simulink model "LUT_liver_pancreas_25"  (R2023b)
settings: Solver=FixedStepAuto  StartTime=0  StopTime=10.1  FixedStep=Timegap  RelTol=1e-3
model workspace (MAT data in the model file):
  T1_input = 1.34
(part 2 of 3)

== system LUT_liver_pancreas_25/If Action Subsystem6/If Action Subsystem1/If Action Subsystem6/If Action Subsystem3 ==
  In1 : Inport
  Action Port : ActionPort  ActionPortLabel=elseif( u1 >= 1.025)
  LUT 1.03RR : Lookup_n-D  NumberOfTableDimensions=1  BreakpointsForDimension1=[403.1578;512.2788;611.2464;710.3985;809.5013;908.5484;1007.552;1106.523;1205.471;1304.4;1403.315;1502.219;1601.114;1700.001;1798.878;1897.738;1996.552]  Table=[400;500;600;700;800;900;1000;1100;1200;1300;1400;1500;1600;1700;1800;1900;2000]  InternalRulePriority=Speed  RndMeth=Simplest
  Out1 : Outport
  wires:
  In1/1 -> LUT 1.03RR/1
  LUT 1.03RR/1 -> Out1/1

== system LUT_liver_pancreas_25/If Action Subsystem6/If Action Subsystem1/If Action Subsystem6/If Action Subsystem4 ==
  In1 : Inport
  Action Port : ActionPort  ActionPortLabel=elseif( u1 >= 1.035)
  LUT 1.04RR : Lookup_n-D  NumberOfTableDimensions=1  BreakpointsForDimension1=[403.058;512.1074;611.0037;710.0774;809.0975;908.0593;1006.976;1105.859;1204.716;1303.555;1402.38;1501.193;1599.996;1698.791;1797.577;1896.347;1995.079]  Table=[400;500;600;700;800;900;1000;1100;1200;1300;1400;1500;1600;1700;1800;1900;2000]  InternalRulePriority=Speed  RndMeth=Simplest
  Out1 : Outport
  wires:
  In1/1 -> LUT 1.04RR/1
  LUT 1.04RR/1 -> Out1/1

== system LUT_liver_pancreas_25/If Action Subsystem6/If Action Subsystem1/If Action Subsystem6/If Action Subsystem5 ==
  In1 : Inport
  Action Port : ActionPort  ActionPortLabel=elseif( u1 >= 1.055)
  LUT 1.06RR : Lookup_n-D  NumberOfTableDimensions=1  BreakpointsForDimension1=[402.866;511.7786;610.5383;709.461;808.3215;907.1183;1005.866;1104.578;1203.263;1301.927;1400.576;1499.212;1597.839;1696.456;1795.064;1893.659;1992.228]  Table=[400;500;600;700;800;900;1000;1100;1200;1300;1400;1500;1600;1700;1800;1900;2000]  InternalRulePriority=Speed  RndMeth=Simplest
  Out1 : Outport
  wires:
  In1/1 -> LUT 1.06RR/1
  LUT 1.06RR/1 -> Out1/1

== system LUT_liver_pancreas_25/If Action Subsystem6/If Action Subsystem1/If Action Subsystem6/If Action Subsystem6 ==
  In1 : Inport
  Action Port : ActionPort  ActionPortLabel=elseif( u1 >= 1.045)
  LUT 1.05RR : Lookup_n-D  NumberOfTableDimensions=1  BreakpointsForDimension1=[402.9608;511.9407;610.7678;709.765;808.7044;907.5827;1006.414;1105.21;1203.981;1302.731;1401.467;1500.191;1598.905;1697.61;1796.306;1894.988;1993.638]  Table=[400;500;600;700;800;900;1000;1100;1200;1300;1400;1500;1600;1700;1800;1900;2000]  InternalRulePriority=Speed  RndMeth=Simplest
  Out1 : Outport
  wires:
  In1/1 -> LUT 1.05RR/1
  LUT 1.05RR/1 -> Out1/1

== system LUT_liver_pancreas_25/If Action Subsystem6/If Action Subsystem1/If Action Subsystem6/If Action Subsystem7 ==
  In1 : Inport
  Action Port : ActionPort  ActionPortLabel=elseif( u1 >= 1.065)
  LUT 1.07RR : Lookup_n-D  NumberOfTableDimensions=1  BreakpointsForDimension1=[402.7736;511.6208;610.315;709.165;807.9485;906.6656;1005.332;1103.961;1202.562;1301.142;1399.706;1498.257;1596.797;1695.328;1793.85;1892.36;1990.847]  Table=[400;500;600;700;800;900;1000;1100;1200;1300;1400;1500;1600;1700;1800;1900;2000]  InternalRulePriority=Speed  RndMeth=Simplest
  Out1 : Outport
  wires:
  In1/1 -> LUT 1.07RR/1
  LUT 1.07RR/1 -> Out1/1

== system LUT_liver_pancreas_25/If Action Subsystem6/If Action Subsystem1/If Action Subsystem6/If Action Subsystem8 ==
  In1 : Inport
  Action Port : ActionPort  ActionPortLabel=elseif(u1 >= 1.075)
  LUT 1.08RR : Lookup_n-D  NumberOfTableDimensions=1  BreakpointsForDimension1=[402.6834;511.4673;610.0977;708.8767;807.585;906.2243;1004.811;1103.359;1201.878;1300.375;1398.855;1497.323;1595.779;1694.226;1792.664;1891.09;1989.496]  Table=[400;500;600;700;800;900;1000;1100;1200;1300;1400;1500;1600;1700;1800;1900;2000]  InternalRulePriority=Speed  RndMeth=Simplest
  Out1 : Outport
  wires:
  In1/1 -> LUT 1.08RR/1
  LUT 1.08RR/1 -> Out1/1

== system LUT_liver_pancreas_25/If Action Subsystem6/If Action Subsystem1/If Action Subsystem6/If Action Subsystem9 ==
  In1 : Inport
  Action Port : ActionPort  ActionPortLabel=if(u1 >= 1.085)
  LUT 1.09RR : Lookup_n-D  NumberOfTableDimensions=1  BreakpointsForDimension1=[402.5954;511.3177;609.886;708.5958;807.2308;905.7938;1004.302;1102.771;1201.21;1299.626;1398.025;1496.41;1594.784;1693.149;1791.504;1889.848;1988.174]  Table=[400;500;600;700;800;900;1000;1100;1200;1300;1400;1500;1600;1700;1800;1900;2000]  InternalRulePriority=Speed  RndMeth=Simplest
  Out1 : Outport
  wires:
  In1/1 -> LUT 1.09RR/1
  LUT 1.09RR/1 -> Out1/1

== system LUT_liver_pancreas_25/If Action Subsystem6/If Action Subsystem1/If Action Subsystem7/If Action Subsystem1 ==
  In1 : Inport
  Action Port : ActionPort  ActionPortLabel=elseif( u1 >= 1.215)
  LUT 1.22RR : Lookup_n-D  NumberOfTableDimensions=1  BreakpointsForDimension1=[401.6092;509.6767;607.5712;705.5178;803.3346;901.0436;998.6735;1096.246;1193.776;1291.274;1388.747;1486.201;1583.64;1681.066;1778.481;1875.887;1973.283]  Table=[400;500;600;700;800;900;1000;1100;1200;1300;1400;1500;1600;1700;1800;1900;2000]  InternalRulePriority=Speed  RndMeth=Simplest
  Out1 : Outport
  wires:
  In1/1 -> LUT 1.22RR/1
  LUT 1.22RR/1 -> Out1/1

== system LUT_liver_pancreas_25/If Action Subsystem6/If Action Subsystem1/If Action Subsystem7/If Action Subsystem10 ==
  In1 : Inport
  Action Port : ActionPort  ActionPortLabel=elseif( u1 >= 1.205)
  LUT 1.21RR : Lookup_n-D  NumberOfTableDimensions=1  BreakpointsForDimension1=[401.6763;509.7858;607.7244;705.7218;803.5935;901.3603;999.0498;1096.683;1194.275;1291.836;1389.373;1486.891;1584.394;1681.884;1779.364;1876.834;1974.294]  Table=[400;500;600;700;800;900;1000;1100;1200;1300;1400;1500;1600;1700;1800;1900;2000]  InternalRulePriority=Speed  RndMeth=Simplest
  Out1 : Outport
  wires:
  In1/1 -> LUT 1.21RR/1
  LUT 1.21RR/1 -> Out1/1

== system LUT_liver_pancreas_25/If Action Subsystem6/If Action Subsystem1/If Action Subsystem7/If Action Subsystem2 ==
  In1 : Inport
  Action Port : ActionPort  ActionPortLabel=else
  LUT 1.20RR : Lookup_n-D  NumberOfTableDimensions=1  BreakpointsForDimension1=[401.7447;509.8975;607.8813;705.9306;803.8585;901.6842;999.4346;1097.13;1194.785;1292.41;1390.012;1487.594;1585.163;1682.719;1780.264;1877.8;1975.326]  Table=[400;500;600;700;800;900;1000;1100;1200;1300;1400;1500;1600;1700;1800;1900;2000]  InternalRulePriority=Speed  RndMeth=Simplest
  Out1 : Outport
  wires:
  In1/1 -> LUT 1.20RR/1
  LUT 1.20RR/1 -> Out1/1

== system LUT_liver_pancreas_25/If Action Subsystem6/If Action Subsystem1/If Action Subsystem7/If Action Subsystem3 ==
  In1 : Inport
  Action Port : ActionPort  ActionPortLabel=elseif( u1 >= 1.225)
  LUT 1.23RR : Lookup_n-D  NumberOfTableDimensions=1  BreakpointsForDimension1=[401.5433;509.5699;607.4215;705.3185;803.0815;900.7339;998.3054;1095.818;1193.287;1290.723;1388.135;1485.526;1582.902;1680.265;1777.616;1874.958;1972.291]  Table=[400;500;600;700;800;900;1000;1100;1200;1300;1400;1500;1600;1700;1800;1900;2000]  InternalRulePriority=Speed  RndMeth=Simplest
  Out1 : Outport
  wires:
  In1/1 -> LUT 1.23RR/1
  LUT 1.23RR/1 -> Out1/1

== system LUT_liver_pancreas_25/If Action Subsystem6/If Action Subsystem1/If Action Subsystem7/If Action Subsystem4 ==
  In1 : Inport
  Action Port : ActionPort  ActionPortLabel=elseif( u1 >= 1.235)
  LUT 1.24RR : Lookup_n-D  NumberOfTableDimensions=1  BreakpointsForDimension1=[401.4785;509.4655;607.2752;705.1238;802.8342;900.4312;997.9452;1095.399;1192.808;1290.184;1387.534;1484.864;1582.178;1679.479;1776.768;1874.048;1971.318]  Table=[400;500;600;700;800;900;1000;1100;1200;1300;1400;1500;1600;1700;1800;1900;2000]  InternalRulePriority=Speed  RndMeth=Simplest
  Out1 : Outport
  wires:
  In1/1 -> LUT 1.24RR/1
  LUT 1.24RR/1 -> Out1/1

== system LUT_liver_pancreas_25/If Action Subsystem6/If Action Subsystem1/If Action Subsystem7/If Action Subsystem5 ==
  In1 : Inport
  Action Port : ActionPort  ActionPortLabel=elseif( u1 >= 1.255)
  LUT 1.26RR : Lookup_n-D  NumberOfTableDimensions=1  BreakpointsForDimension1=[401.3524;509.2634;606.9926;704.7476;802.3561;899.8455;997.2481;1094.588;1191.881;1289.139;1386.37;1483.58;1580.774;1677.953;1775.121;1872.279;1969.428]  Table=[400;500;600;700;800;900;1000;1100;1200;1300;1400;1500;1600;1700;1800;1900;2000]  InternalRulePriority=Speed  RndMeth=Simplest
  Out1 : Outport
  wires:
  In1/1 -> LUT 1.26RR/1
  LUT 1.26RR/1 -> Out1/1

== system LUT_liver_pancreas_25/If Action Subsystem6/If Action Subsystem1/If Action Subsystem7/If Action Subsystem6 ==
  In1 : Inport
  Action Port : ActionPort  ActionPortLabel=elseif( u1 >= 1.245)
  LUT 1.25RR : Lookup_n-D  NumberOfTableDimensions=1  BreakpointsForDimension1=[401.4149;509.3633;607.1323;704.9335;802.5924;900.1351;997.5929;1094.989;1192.34;1289.656;1386.946;1484.216;1581.469;1678.709;1775.937;1873.155;1970.364]  Table=[400;500;600;700;800;900;1000;1100;1200;1300;1400;1500;1600;1700;1800;1900;2000]  InternalRulePriority=Speed  RndMeth=Simplest
  Out1 : Outport
  wires:
  In1/1 -> LUT 1.25RR/1
  LUT 1.25RR/1 -> Out1/1

== system LUT_liver_pancreas_25/If Action Subsystem6/If Action Subsystem1/If Action Subsystem7/If Action Subsystem7 ==
  In1 : Inport
  Action Port : ActionPort  ActionPortLabel=elseif( u1 >= 1.265)
  LUT 1.27RR : Lookup_n-D  NumberOfTableDimensions=1  BreakpointsForDimension1=[401.291;509.1656;606.856;704.5658;802.125;899.5622;996.9107;1094.195;1191.431;1288.632;1385.806;1482.957;1580.092;1677.213;1774.322;1871.42;1968.51]  Table=[400;500;600;700;800;900;1000;1100;1200;1300;1400;1500;1600;1700;1800;1900;2000]  InternalRulePriority=Speed  RndMeth=Simplest
  Out1 : Outport
  wires:
  In1/1 -> LUT 1.27RR/1
  LUT 1.27RR/1 -> Out1/1

== system LUT_liver_pancreas_25/If Action Subsystem6/If Action Subsystem1/If Action Subsystem7/If Action Subsystem8 ==
  In1 : Inport
  Action Port : ActionPort  ActionPortLabel=elseif(u1 >= 1.275)
  LUT 1.28RR : Lookup_n-D  NumberOfTableDimensions=1  BreakpointsForDimension1=[401.2306;509.0698;606.7226;704.3882;801.899;899.2851;996.5805;1093.81;1190.991;1288.136;1385.252;1482.347;1579.424;1676.486;1773.537;1870.577;1967.608]  Table=[400;500;600;700;800;900;1000;1100;1200;1300;1400;1500;1600;1700;1800;1900;2000]  InternalRulePriority=Speed  RndMeth=Simplest
  Out1 : Outport
  wires:
  In1/1 -> LUT 1.28RR/1
  LUT 1.28RR/1 -> Out1/1

== system LUT_liver_pancreas_25/If Action Subsystem6/If Action Subsystem1/If Action Subsystem7/If Action Subsystem9 ==
  In1 : Inport
  Action Port : ActionPort  ActionPortLabel=if(u1 >= 1.285)
  LUT 1.29RR : Lookup_n-D  NumberOfTableDimensions=1  BreakpointsForDimension1=[401.1711;508.9761;606.5921;704.2145;801.678;899.014;996.2573;1093.433;1190.56;1287.649;1384.71;1481.748;1578.768;1675.774;1772.767;1869.751;1966.724]  Table=[400;500;600;700;800;900;1000;1100;1200;1300;1400;1500;1600;1700;1800;1900;2000]  InternalRulePriority=Speed  RndMeth=Simplest
  Out1 : Outport
  wires:
  In1/1 -> LUT 1.29RR/1
  LUT 1.29RR/1 -> Out1/1

== system LUT_liver_pancreas_25/If Action Subsystem6/If Action Subsystem1/If Action Subsystem8/If Action Subsystem1 ==
  In1 : Inport
  Action Port : ActionPort  ActionPortLabel=elseif( u1 >= 1.315)
  LUT 1.32RR : Lookup_n-D  NumberOfTableDimensions=1  BreakpointsForDimension1=[400.9985;508.7063;606.2176;703.7164;801.0438;898.2352;995.328;1092.349;1189.318;1286.247;1383.146;1480.021;1576.876;1673.717;1770.544;1867.361;1964.168]  Table=[400;500;600;700;800;900;1000;1100;1200;1300;1400;1500;1600;1700;1800;1900;2000]  InternalRulePriority=Speed  RndMeth=Simplest
  Out1 : Outport
  wires:
  In1/1 -> LUT 1.32RR/1
  LUT 1.32RR/1 -> Out1/1

== system LUT_liver_pancreas_25/If Action Subsystem6/If Action Subsystem1/If Action Subsystem8/If Action Subsystem10 ==
  In1 : Inport
  Action Port : ActionPort  ActionPortLabel=elseif( u1 >= 1.305)
  LUT 1.31RR : Lookup_n-D  NumberOfTableDimensions=1  BreakpointsForDimension1=[401.0551;508.7943;606.3397;703.8787;801.2505;898.4892;995.6313;1092.703;1189.724;1286.705;1383.657;1480.585;1577.495;1674.389;1771.272;1868.143;1965.004]  Table=[400;500;600;700;800;900;1000;1100;1200;1300;1400;1500;1600;1700;1800;1900;2000]  InternalRulePriority=Speed  RndMeth=Simplest
  Out1 : Outport
  wires:
  In1/1 -> LUT 1.31RR/1
  LUT 1.31RR/1 -> Out1/1

== system LUT_liver_pancreas_25/If Action Subsystem6/If Action Subsystem1/If Action Subsystem8/If Action Subsystem2 ==
  In1 : Inport
  Action Port : ActionPort  ActionPortLabel=else
  LUT 1.30RR : Lookup_n-D  NumberOfTableDimensions=1  BreakpointsForDimension1=[401.1126;508.8843;606.4645;704.0447;801.4619;898.7488;995.941;1093.065;1190.137;1287.172;1384.178;1481.161;1578.125;1675.075;1772.012;1868.939;1965.856]  Table=[400;500;600;700;800;900;1000;1100;1200;1300;1400;1500;1600;1700;1800;1900;2000]  InternalRulePriority=Speed  RndMeth=Simplest
  Out1 : Outport
  wires:
  In1/1 -> LUT 1.30RR/1
  LUT 1.30RR/1 -> Out1/1

== system LUT_liver_pancreas_25/If Action Subsystem6/If Action Subsystem1/If Action Subsystem8/If Action Subsystem3 ==
  In1 : Inport
  Action Port : ActionPort  ActionPortLabel=elseif( u1 >= 1.325)
  LUT 1.33RR : Lookup_n-D  NumberOfTableDimensions=1  BreakpointsForDimension1=[400.9427;508.62;606.0983;703.5577;800.8415;897.9866;995.0311;1092.003;1188.921;1285.798;1382.645;1479.467;1576.27;1673.057;1769.831;1866.594;1963.347]  Table=[400;500;600;700;800;900;1000;1100;1200;1300;1400;1500;1600;1700;1800;1900;2000]  InternalRulePriority=Speed  RndMeth=Simplest
  Out1 : Outport
  wires:
  In1/1 -> LUT 1.33RR/1
  LUT 1.33RR/1 -> Out1/1

== system LUT_liver_pancreas_25/If Action Subsystem6/If Action Subsystem1/If Action Subsystem8/If Action Subsystem4 ==
  In1 : Inport
  Action Port : ActionPort  ActionPortLabel=elseif( u1 >= 1.335)
  LUT 1.34RR : Lookup_n-D  NumberOfTableDimensions=1  BreakpointsForDimension1=[400.8878;508.5354;605.9815;703.4024;800.6436;897.7433;994.7404;1091.663;1188.531;1285.358;1382.153;1478.924;1575.674;1672.409;1769.131;1865.841;1962.541]  Table=[400;500;600;700;800;900;1000;1100;1200;1300;1400;1500;1600;1700;1800;1900;2000]  InternalRulePriority=Speed  RndMeth=Simplest
  Out1 : Outport
  wires:
  In1/1 -> LUT 1.34RR/1
  LUT 1.34RR/1 -> Out1/1

== system LUT_liver_pancreas_25/If Action Subsystem6/If Action Subsystem1/If Action Subsystem8/If Action Subsystem5 ==
  In1 : Inport
  Action Port : ActionPort  ActionPortLabel=elseif( u1 >= 1.355)
  LUT 1.36RR : Lookup_n-D  NumberOfTableDimensions=1  BreakpointsForDimension1=[400.7805;508.3714;605.7554;703.102;800.2606;897.272;994.1769;1091.005;1187.775;1284.503;1381.198;1477.868;1574.517;1671.149;1767.768;1864.375;1960.972]  Table=[400;500;600;700;800;900;1000;1100;1200;1300;1400;1500;1600;1700;1800;1900;2000]  InternalRulePriority=Speed  RndMeth=Simplest
  Out1 : Outport
  wires:
  In1/1 -> LUT 1.36RR/1
  LUT 1.36RR/1 -> Out1/1

== system LUT_liver_pancreas_25/If Action Subsystem6/If Action Subsystem1/If Action Subsystem8/If Action Subsystem6 ==
  In1 : Inport
  Action Port : ActionPort  ActionPortLabel=elseif( u1 >= 1.345)
  LUT 1.35RR : Lookup_n-D  NumberOfTableDimensions=1  BreakpointsForDimension1=[400.8337;508.4526;605.8672;703.2505;800.4501;897.5052;994.4557;1091.331;1188.15;1284.926;1381.671;1478.391;1575.09;1671.773;1768.443;1865.101;1961.75]  Table=[400;500;600;700;800;900;1000;1100;1200;1300;1400;1500;1600;1700;1800;1900;2000]  InternalRulePriority=Speed  RndMeth=Simplest
  Out1 : Outport
  wires:
  In1/1 -> LUT 1.35RR/1
  LUT 1.35RR/1 -> Out1/1

== system LUT_liver_pancreas_25/If Action Subsystem6/If Action Subsystem1/If Action Subsystem8/If Action Subsystem7 ==
  In1 : Inport
  Action Port : ActionPort  ActionPortLabel=elseif( u1 >= 1.365)
  LUT 1.37RR : Lookup_n-D  NumberOfTableDimensions=1  BreakpointsForDimension1=[400.728;508.2918;605.646;702.9566;800.0753;897.0438;993.9039;1090.685;1187.409;1284.088;1380.735;1477.355;1573.954;1670.537;1767.105;1863.662;1960.209]  Table=[400;500;600;700;800;900;1000;1100;1200;1300;1400;1500;1600;1700;1800;1900;2000]  InternalRulePriority=Speed  RndMeth=Simplest
  Out1 : Outport
  wires:
  In1/1 -> LUT 1.37RR/1
  LUT 1.37RR/1 -> Out1/1

== system LUT_liver_pancreas_25/If Action Subsystem6/If Action Subsystem1/If Action Subsystem8/If Action Subsystem8 ==
  In1 : Inport
  Action Port : ActionPort  ActionPortLabel=elseif(u1 >= 1.375)
  LUT 1.38RR : Lookup_n-D  NumberOfTableDimensions=1  BreakpointsForDimension1=[400.6763;508.2137;605.539;702.8145;799.8939;896.8204;993.6364;1090.372;1187.049;1283.682;1380.28;1476.852;1573.402;1669.936;1766.455;1862.962;1959.459]  Table=[400;500;600;700;800;900;1000;1100;1200;1300;1400;1500;1600;1700;1800;1900;2000]  InternalRulePriority=Speed  RndMeth=Simplest
  Out1 : Outport
  wires:
  In1/1 -> LUT 1.38RR/1
  LUT 1.38RR/1 -> Out1/1

== system LUT_liver_pancreas_25/If Action Subsystem6/If Action Subsystem1/If Action Subsystem8/If Action Subsystem9 ==
  In1 : Inport
  Action Port : ActionPort  ActionPortLabel=if(u1 >= 1.385)
  LUT 1.39RR : Lookup_n-D  NumberOfTableDimensions=1  BreakpointsForDimension1=[400.6253;508.1372;605.4342;702.6754;799.7164;896.6017;993.3744;1090.066;1186.697;1283.283;1379.834;1476.358;1572.86;1669.345;1765.816;1862.275;1958.723]  Table=[400;500;600;700;800;900;1000;1100;1200;1300;1400;1500;1600;1700;1800;1900;2000]  InternalRulePriority=Speed  RndMeth=Simplest
  Out1 : Outport
  wires:
  In1/1 -> LUT 1.39RR/1
  LUT 1.39RR/1 -> Out1/1

== system LUT_liver_pancreas_25/If Action Subsystem6/If Action Subsystem1/If Action Subsystem9/If Action Subsystem1 ==
  In1 : Inport
  Action Port : ActionPort  ActionPortLabel=elseif( u1 >= 1.415)
  LUT 1.42RR : Lookup_n-D  NumberOfTableDimensions=1  BreakpointsForDimension1=[400.4767;507.9164;605.133;702.2758;799.2063;895.9725;992.6201;1089.182;1185.68;1282.131;1378.545;1474.931;1571.293;1667.638;1763.967;1860.284;1956.59]  Table=[400;500;600;700;800;900;1000;1100;1200;1300;1400;1500;1600;1700;1800;1900;2000]  InternalRulePriority=Speed  RndMeth=Simplest
  Out1 : Outport
  wires:
  In1/1 -> LUT 1.42RR/1
  LUT 1.42RR/1 -> Out1/1

== system LUT_liver_pancreas_25/If Action Subsystem6/If Action Subsystem1/If Action Subsystem9/If Action Subsystem10 ==
  In1 : Inport
  Action Port : ActionPort  ActionPortLabel=elseif( u1 >= 1.405)
  LUT 1.41RR : Lookup_n-D  NumberOfTableDimensions=1  BreakpointsForDimension1=[400.5255;507.9886;605.2312;702.4061;799.3727;896.1778;992.8664;1089.471;1186.012;1282.507;1378.966;1475.397;1571.806;1668.197;1764.572;1860.936;1957.288]  Table=[400;500;600;700;800;900;1000;1100;1200;1300;1400;1500;1600;1700;1800;1900;2000]  InternalRulePriority=Speed  RndMeth=Simplest
  Out1 : Outport
  wires:
  In1/1 -> LUT 1.41RR/1
  LUT 1.41RR/1 -> Out1/1

== system LUT_liver_pancreas_25/If Action Subsystem6/If Action Subsystem1/If Action Subsystem9/If Action Subsystem2 ==
  In1 : Inport
  Action Port : ActionPort  ActionPortLabel=else
  LUT 1.40RR : Lookup_n-D  NumberOfTableDimensions=1  BreakpointsForDimension1=[400.5751;508.0622;605.3316;702.5393;799.5427;896.3875;993.1178;1089.765;1186.351;1282.891;1379.396;1475.873;1572.328;1668.766;1765.189;1861.599;1957.999]  Table=[400;500;600;700;800;900;1000;1100;1200;1300;1400;1500;1600;1700;1800;1900;2000]  InternalRulePriority=Speed  RndMeth=Simplest
  Out1 : Outport
  wires:
  In1/1 -> LUT 1.40RR/1
  LUT 1.40RR/1 -> Out1/1

== system LUT_liver_pancreas_25/If Action Subsystem6/If Action Subsystem1/If Action Subsystem9/If Action Subsystem3 ==
  In1 : Inport
  Action Port : ActionPort  ActionPortLabel=elseif( u1 >= 1.425)
  LUT 1.43RR : Lookup_n-D  NumberOfTableDimensions=1  BreakpointsForDimension1=[400.4285;507.8455;605.0367;702.1483;799.0434;895.7714;992.3788;1088.899;1185.354;1281.762;1378.131;1474.472;1570.79;1667.089;1763.373;1859.643;1955.903]  Table=[400;500;600;700;800;900;1000;1100;1200;1300;1400;1500;1600;1700;1800;1900;2000]  InternalRulePriority=Speed  RndMeth=Simplest
  Out1 : Outport
  wires:
  In1/1 -> LUT 1.43RR/1
  LUT 1.43RR/1 -> Out1/1

== system LUT_liver_pancreas_25/If Action Subsystem6/If Action Subsystem1/If Action Subsystem9/If Action Subsystem4 ==
  In1 : Inport
  Action Port : ActionPort  ActionPortLabel=elseif( u1 >= 1.435)
  LUT 1.44RR : Lookup_n-D  NumberOfTableDimensions=1  BreakpointsForDimension1=[400.381;507.776;604.9425;702.0235;798.884;895.5745;992.1424;1088.621;1185.035;1281.399;1377.726;1474.022;1570.296;1666.55;1762.789;1859.014;1955.229]  Table=[400;500;600;700;800;900;1000;1100;1200;1300;1400;1500;1600;1700;1800;1900;2000]  InternalRulePriority=Speed  RndMeth=Simplest
  Out1 : Outport
  wires:
  In1/1 -> LUT 1.44RR/1
  LUT 1.44RR/1 -> Out1/1

== system LUT_liver_pancreas_25/If Action Subsystem6/If Action Subsystem1/If Action Subsystem9/If Action Subsystem5 ==
  In1 : Inport
  Action Port : ActionPort  ActionPortLabel=elseif( u1 >= 1.455)
  LUT 1.46RR : Lookup_n-D  NumberOfTableDimensions=1  BreakpointsForDimension1=[400.2879;507.6409;604.76;701.7818;798.5751;895.1928;991.6838;1088.083;1184.414;1280.695;1376.936;1473.147;1569.333;1665.5;1761.651;1857.788;1953.914]  Table=[400;500;600;700;800;900;1000;1100;1200;1300;1400;1500;1600;1700;1800;1900;2000]  InternalRulePriority=Speed  RndMeth=Simplest
  Out1 : Outport
  wires:
  In1/1 -> LUT 1.46RR/1
  LUT 1.46RR/1 -> Out1/1

== system LUT_liver_pancreas_25/If Action Subsystem6/If Action Subsystem1/If Action Subsystem9/If Action Subsystem6 ==
  In1 : Inport
  Action Port : ActionPort  ActionPortLabel=elseif( u1 >= 1.445)
  LUT 1.45RR : Lookup_n-D  NumberOfTableDimensions=1  BreakpointsForDimension1=[400.3341;507.7078;604.8503;701.9014;798.7279;895.3816;991.9107;1088.35;1184.722;1281.044;1377.327;1473.581;1569.81;1666.02;1762.215;1858.396;1954.566]  Table=[400;500;600;700;800;900;1000;1100;1200;1300;1400;1500;1600;1700;1800;1900;2000]  InternalRulePriority=Speed  RndMeth=Simplest
  Out1 : Outport
  wires:
  In1/1 -> LUT 1.45RR/1
  LUT 1.45RR/1 -> Out1/1

== system LUT_liver_pancreas_25/If Action Subsystem6/If Action Subsystem1/If Action Subsystem9/If Action Subsystem7 ==
  In1 : Inport
  Action Port : ActionPort  ActionPortLabel=elseif( u1 >= 1.465)
  LUT 1.47RR : Lookup_n-D  NumberOfTableDimensions=1  BreakpointsForDimension1=[400.2422;507.5752;604.6715;701.6648;798.4255;895.0078;991.4613;1087.822;1184.113;1280.353;1376.552;1472.721;1568.865;1664.989;1761.097;1857.191;1953.274]  Table=[400;500;600;700;800;900;1000;1100;1200;1300;1400;1500;1600;1700;1800;1900;2000]  InternalRulePriority=Speed  RndMeth=Simplest
  Out1 : Outport
  wires:
  In1/1 -> LUT 1.47RR/1
  LUT 1.47RR/1 -> Out1/1

== system LUT_liver_pancreas_25/If Action Subsystem6/If Action Subsystem1/If Action Subsystem9/If Action Subsystem8 ==
  In1 : Inport
  Action Port : ActionPort  ActionPortLabel=elseif(u1 >= 1.475)
  LUT 1.48RR : Lookup_n-D  NumberOfTableDimensions=1  BreakpointsForDimension1=[400.1972;507.5108;604.5849;701.5503;798.2791;894.8266;991.2434;1087.565;1183.817;1280.017;1376.176;1472.303;1568.405;1664.487;1760.553;1856.604;1952.644]  Table=[400;500;600;700;800;900;1000;1100;1200;1300;1400;1500;1600;1700;1800;1900;2000]  InternalRulePriority=Speed  RndMeth=Simplest
  Out1 : Outport
  wires:
  In1/1 -> LUT 1.48RR/1
  LUT 1.48RR/1 -> Out1/1

== system LUT_liver_pancreas_25/If Action Subsystem6/If Action Subsystem1/If Action Subsystem9/If Action Subsystem9 ==
  In1 : Inport
  Action Port : ActionPort  ActionPortLabel=if(u1 >= 1.485)
  LUT 1.49RR : Lookup_n-D  NumberOfTableDimensions=1  BreakpointsForDimension1=[400.1527;507.4475;604.5;701.4382;798.1357;894.6491;991.0298;1087.314;1183.527;1279.687;1375.806;1471.893;1567.954;1663.994;1760.018;1856.028;1952.025]  Table=[400;500;600;700;800;900;1000;1100;1200;1300;1400;1500;1600;1700;1800;1900;2000]  InternalRulePriority=Speed  RndMeth=Simplest
  Out1 : Outport
  wires:
  In1/1 -> LUT 1.49RR/1
  LUT 1.49RR/1 -> Out1/1

== system LUT_liver_pancreas_25/If Action Subsystem6/If Action Subsystem2/If Action Subsystem5/If Action Subsystem1 ==
  In1 : Inport
  Action Port : ActionPort  ActionPortLabel=elseif( u1 >= 1.615)
  LUT 1.62RR : Lookup_n-D  NumberOfTableDimensions=1  BreakpointsForDimension1=[399.6228;506.7204;603.542;700.1784;796.523;892.6467;988.6108;1084.459;1180.221;1275.919;1371.567;1467.176;1562.753;1658.306;1753.839;1849.355;1944.857]  Table=[400;500;600;700;800;900;1000;1100;1200;1300;1400;1500;1600;1700;1800;1900;2000]  InternalRulePriority=Speed  RndMeth=Simplest
  Out1 : Outport
  wires:
  In1/1 -> LUT 1.62RR/1
  LUT 1.62RR/1 -> Out1/1

== system LUT_liver_pancreas_25/If Action Subsystem6/If Action Subsystem2/If Action Subsystem5/If Action Subsystem10 ==
  In1 : Inport
  Action Port : ActionPort  ActionPortLabel=elseif( u1>= 1.605)
  LUT 1.61RR : Lookup_n-D  NumberOfTableDimensions=1  BreakpointsForDimension1=[399.6606;506.7706;603.607;700.2634;796.632;892.7824;988.7753;1084.654;1180.448;1276.178;1371.858;1467.501;1563.113;1658.7;1754.268;1849.818;1945.355]  Table=[400;500;600;700;800;900;1000;1100;1200;1300;1400;1500;1600;1700;1800;1900;2000]  InternalRulePriority=Speed  RndMeth=Simplest
  Out1 : Outport
  wires:
  In1/1 -> LUT 1.61RR/1
  LUT 1.61RR/1 -> Out1/1

== system LUT_liver_pancreas_25/If Action Subsystem6/If Action Subsystem2/If Action Subsystem5/If Action Subsystem2 ==
  In1 : Inport
  Action Port : ActionPort  ActionPortLabel=else
  LUT 1.60RR : Lookup_n-D  NumberOfTableDimensions=1  BreakpointsForDimension1=[399.699;506.8217;603.6734;700.3504;796.7433;892.9209;988.9432;1084.853;1180.678;1276.441;1372.156;1467.832;1563.479;1659.101;1754.703;1850.289;1945.862]  Table=[400;500;600;700;800;900;1000;1100;1200;1300;1400;1500;1600;1700;1800;1900;2000]  InternalRulePriority=Speed  RndMeth=Simplest
  Out1 : Outport
  wires:
  In1/1 -> LUT 1.60RR/1
  LUT 1.60RR/1 -> Out1/1

== system LUT_liver_pancreas_25/If Action Subsystem6/If Action Subsystem2/If Action Subsystem5/If Action Subsystem3 ==
  In1 : Inport
  Action Port : ActionPort  ActionPortLabel=elseif( u1 >= 1.625)
  LUT 1.63RR : Lookup_n-D  NumberOfTableDimensions=1  BreakpointsForDimension1=[399.5853;506.671;603.4782;700.095;796.4163;892.5137;988.4495;1084.268;1179.999;1275.665;1371.28;1466.856;1562.4;1657.919;1753.418;1848.899;1944.366]  Table=[400;500;600;700;800;900;1000;1100;1200;1300;1400;1500;1600;1700;1800;1900;2000]  InternalRulePriority=Speed  RndMeth=Simplest
  Out1 : Outport
  wires:
  In1/1 -> LUT 1.63RR/1
  LUT 1.63RR/1 -> Out1/1

== system LUT_liver_pancreas_25/If Action Subsystem6/If Action Subsystem2/If Action Subsystem5/If Action Subsystem4 ==
  In1 : Inport
  Action Port : ActionPort  ActionPortLabel=elseif( u1 >= 1.635)
  LUT 1.64RR : Lookup_n-D  NumberOfTableDimensions=1  BreakpointsForDimension1=[399.5483;506.6225;603.4157;700.0135;796.3117;892.3834;988.2914;1084.08;1179.781;1275.415;1370.998;1466.542;1562.053;1657.538;1753.003;1848.451;1943.883]  Table=[400;500;600;700;800;900;1000;1100;1200;1300;1400;1500;1600;1700;1800;1900;2000]  InternalRulePriority=Speed  RndMeth=Simplest
  Out1 : Outport
  wires:
  In1/1 -> LUT 1.64RR/1
  LUT 1.64RR/1 -> Out1/1

== system LUT_liver_pancreas_25/If Action Subsystem6/If Action Subsystem2/If Action Subsystem5/If Action Subsystem5 ==
  In1 : Inport
  Action Port : ActionPort  ActionPortLabel=elseif( u1 >= 1.655)
  LUT 1.66RR : Lookup_n-D  NumberOfTableDimensions=1  BreakpointsForDimension1=[399.4756;506.5279;603.2945;699.8554;796.1092;892.1308;987.9845;1083.716;1179.357;1274.93;1370.45;1465.929;1561.376;1656.796;1752.195;1847.575;1942.941]  Table=[400;500;600;700;800;900;1000;1100;1200;1300;1400;1500;1600;1700;1800;1900;2000]  InternalRulePriority=Speed  RndMeth=Simplest
  Out1 : Outport
  wires:
  In1/1 -> LUT 1.66RR/1
  LUT 1.66RR/1 -> Out1/1

== system LUT_liver_pancreas_25/If Action Subsystem6/If Action Subsystem2/If Action Subsystem5/If Action Subsystem6 ==
  In1 : Inport
  Action Port : ActionPort  ActionPortLabel=elseif( u1 >= 1.645)
  LUT 1.65RR : Lookup_n-D  NumberOfTableDimensions=1  BreakpointsForDimension1=[399.5117;506.5748;603.3545;699.9336;796.2094;892.2558;988.1364;1083.896;1179.567;1275.17;1370.722;1466.233;1561.711;1657.164;1752.596;1848.009;1943.409]  Table=[400;500;600;700;800;900;1000;1100;1200;1300;1400;1500;1600;1700;1800;1900;2000]  InternalRulePriority=Speed  RndMeth=Simplest
  Out1 : Outport
  wires:
  In1/1 -> LUT 1.65RR/1
  LUT 1.65RR/1 -> Out1/1

== system LUT_liver_pancreas_25/If Action Subsystem6/If Action Subsystem2/If Action Subsystem5/If Action Subsystem7 ==
  In1 : Inport
  Action Port : ActionPort  ActionPortLabel=elseif( u1 >= 1.665)
  LUT 1.67RR : Lookup_n-D  NumberOfTableDimensions=1  BreakpointsForDimension1=[399.4398;506.4817;603.2356;699.7788;796.0111;892.0083;987.8356;1083.539;1179.151;1274.694;1370.183;1465.631;1561.046;1656.434;1751.8;1847.148;1942.482]  Table=[400;500;600;700;800;900;1000;1100;1200;1300;1400;1500;1600;1700;1800;1900;2000]  InternalRulePriority=Speed  RndMeth=Simplest
  Out1 : Outport
  wires:
  In1/1 -> LUT 1.67RR/1
  LUT 1.67RR/1 -> Out1/1

== system LUT_liver_pancreas_25/If Action Subsystem6/If Action Subsystem2/If Action Subsystem5/If Action Subsystem8 ==
  In1 : Inport
  Action Port : ActionPort  ActionPortLabel=elseif(u1 >= 1.675)
  LUT 1.68RR : Lookup_n-D  NumberOfTableDimensions=1  BreakpointsForDimension1=[399.4045;506.4364;603.1779;699.7038;795.915;891.8883;987.6896;1083.366;1178.949;1274.462;1369.921;1465.338;1560.722;1656.078;1751.412;1846.728;1942.029]  Table=[400;500;600;700;800;900;1000;1100;1200;1300;1400;1500;1600;1700;1800;1900;2000]  InternalRulePriority=Speed  RndMeth=Simplest
  Out1 : Outport
  wires:
  In1/1 -> LUT 1.68RR/1
  LUT 1.68RR/1 -> Out1/1

== system LUT_liver_pancreas_25/If Action Subsystem6/If Action Subsystem2/If Action Subsystem5/If Action Subsystem9 ==
  In1 : Inport
  Action Port : ActionPort  ActionPortLabel=if(u1 >= 1.685)
  LUT 1.69RR : Lookup_n-D  NumberOfTableDimensions=1  BreakpointsForDimension1=[399.3695;506.3918;603.1214;699.6304;795.8209;891.7708;987.5466;1083.196;1178.75;1274.234;1369.664;1465.05;1560.403;1655.728;1751.031;1846.315;1941.584]  Table=[400;500;600;700;800;900;1000;1100;1200;1300;1400;1500;1600;1700;1800;1900;2000]  InternalRulePriority=Speed  RndMeth=Simplest
  Out1 : Outport
  wires:
  In1/1 -> LUT 1.69RR/1
  LUT 1.69RR/1 -> Out1/1

== system LUT_liver_pancreas_25/If Action Subsystem6/If Action Subsystem2/If Action Subsystem6/If Action Subsystem1 ==
  In1 : Inport
  Action Port : ActionPort  ActionPortLabel=elseif( u1 >= 1.515)
  LUT 1.52RR : Lookup_n-D  NumberOfTableDimensions=1  BreakpointsForDimension1=[400.0228;507.2644;604.2558;701.1159;797.7234;894.1383;990.4143;1086.589;1182.69;1278.735;1374.737;1470.705;1566.646;1662.566;1758.468;1854.355;1950.231]  Table=[400;500;600;700;800;900;1000;1100;1200;1300;1400;1500;1600;1700;1800;1900;2000]  InternalRulePriority=Speed  RndMeth=Simplest
  Out1 : Outport
  wires:
  In1/1 -> LUT 1.52RR/1
  LUT 1.52RR/1 -> Out1/1

== system LUT_liver_pancreas_25/If Action Subsystem6/If Action Subsystem2/If Action Subsystem6/If Action Subsystem10 ==
  In1 : Inport
  Action Port : ActionPort  ActionPortLabel=elseif( u1 >= 1.505)
  LUT 1.51RR : Lookup_n-D  NumberOfTableDimensions=1  BreakpointsForDimension1=[400.0655;507.3243;604.3355;701.2211;797.858;894.3051;990.6153;1086.826;1182.964;1279.046;1375.087;1471.094;1567.074;1663.034;1758.976;1854.903;1950.819]  Table=[400;500;600;700;800;900;1000;1100;1200;1300;1400;1500;1600;1700;1800;1900;2000]  InternalRulePriority=Speed  RndMeth=Simplest
  Out1 : Outport
  wires:
  In1/1 -> LUT 1.51RR/1
  LUT 1.51RR/1 -> Out1/1

== system LUT_liver_pancreas_25/If Action Subsystem6/If Action Subsystem2/If Action Subsystem6/If Action Subsystem2 ==
  In1 : Inport
  Action Port : ActionPort  ActionPortLabel=else
  LUT 1.50RR : Lookup_n-D  NumberOfTableDimensions=1  BreakpointsForDimension1=[400.1089;507.3853;604.4169;701.3285;797.9954;894.4753;990.8205;1087.068;1183.243;1279.364;1375.443;1471.489;1567.51;1663.51;1759.492;1855.461;1951.417]  Table=[400;500;600;700;800;900;1000;1100;1200;1300;1400;1500;1600;1700;1800;1900;2000]  InternalRulePriority=Speed  RndMeth=Simplest
  Out1 : Outport
  wires:
  In1/1 -> LUT 1.50RR/1
  LUT 1.50RR/1 -> Out1/1

== system LUT_liver_pancreas_25/If Action Subsystem6/If Action Subsystem2/If Action Subsystem6/If Action Subsystem3 ==
  In1 : Inport
  Action Port : ActionPort  ActionPortLabel=elseif( u1 >= 1.525)
  LUT 1.53RR : Lookup_n-D  NumberOfTableDimensions=1  BreakpointsForDimension1=[399.9805;507.2055;604.1777;701.013;797.5917;893.9749;990.2172;1086.357;1182.422;1278.429;1374.393;1470.323;1566.225;1662.106;1757.969;1853.817;1949.652]  Table=[400;500;600;700;800;900;1000;1100;1200;1300;1400;1500;1600;1700;1800;1900;2000]  InternalRulePriority=Speed  RndMeth=Simplest
  Out1 : Outport
  wires:
  In1/1 -> LUT 1.53RR/1
  LUT 1.53RR/1 -> Out1/1

== system LUT_liver_pancreas_25/If Action Subsystem6/If Action Subsystem2/If Action Subsystem6/If Action Subsystem4 ==
  In1 : Inport
  Action Port : ActionPort  ActionPortLabel=elseif( u1 >= 1.535)
  LUT 1.54RR : Lookup_n-D  NumberOfTableDimensions=1  BreakpointsForDimension1=[399.9388;507.1478;604.1012;700.9122;797.4627;893.8149;990.0241;1086.129;1182.158;1278.129;1374.056;1469.948;1565.812;1661.654;1757.478;1853.287;1949.083]  Table=[400;500;600;700;800;900;1000;1100;1200;1300;1400;1500;1600;1700;1800;1900;2000]  InternalRulePriority=Speed  RndMeth=Simplest
  Out1 : Outport
  wires:
  In1/1 -> LUT 1.54RR/1
  LUT 1.54RR/1 -> Out1/1

== system LUT_liver_pancreas_25/If Action Subsystem6/If Action Subsystem2/If Action Subsystem6/If Action Subsystem5 ==
  In1 : Inport
  Action Port : ActionPort  ActionPortLabel=elseif( u1 >= 1.555)
  LUT 1.56RR : Lookup_n-D  NumberOfTableDimensions=1  BreakpointsForDimension1=[399.8569;507.0352;603.9527;700.7169;797.2127;893.5046;989.6493;1085.687;1181.646;1277.546;1373.399;1469.217;1565.007;1660.774;1756.522;1852.254;1947.974]  Table=[400;500;600;700;800;900;1000;1100;1200;1300;1400;1500;1600;1700;1800;1900;2000]  InternalRulePriority=Speed  RndMeth=Simplest
  Out1 : Outport
  wires:
  In1/1 -> LUT 1.56RR/1
  LUT 1.56RR/1 -> Out1/1

== system LUT_liver_pancreas_25/If Action Subsystem6/If Action Subsystem2/If Action Subsystem6/If Action Subsystem6 ==
  In1 : Inport
  Action Port : ActionPort  ActionPortLabel=elseif( u1 >= 1.545)
  LUT 1.55RR : Lookup_n-D  NumberOfTableDimensions=1  BreakpointsForDimension1=[399.8976;507.091;604.0262;700.8135;797.3364;893.6581;989.8348;1085.906;1181.9;1277.835;1373.725;1469.579;1565.406;1661.21;1756.996;1852.766;1948.524]  Table=[400;500;600;700;800;900;1000;1100;1200;1300;1400;1500;1600;1700;1800;1900;2000]  InternalRulePriority=Speed  RndMeth=Simplest
  Out1 : Outport
  wires:
  In1/1 -> LUT 1.55RR/1
  LUT 1.55RR/1 -> Out1/1

== system LUT_liver_pancreas_25/If Action Subsystem6/If Action Subsystem2/If Action Subsystem6/If Action Subsystem7 ==
  In1 : Inport
  Action Port : ActionPort  ActionPortLabel=elseif( u1 >= 1.565)
  LUT 1.57RR : Lookup_n-D  NumberOfTableDimensions=1  BreakpointsForDimension1=[399.8167;506.9804;603.8807;700.6224;797.0917;893.3541;989.4674;1085.472;1181.397;1277.262;1373.08;1468.862;1564.615;1660.345;1756.056;1851.751;1947.433]  Table=[400;500;600;700;800;900;1000;1100;1200;1300;1400;1500;1600;1700;1800;1900;2000]  InternalRulePriority=Speed  RndMeth=Simplest
  Out1 : Outport
  wires:
  In1/1 -> LUT 1.57RR/1
  LUT 1.57RR/1 -> Out1/1

== system LUT_liver_pancreas_25/If Action Subsystem6/If Action Subsystem2/If Action Subsystem6/If Action Subsystem8 ==
  In1 : Inport
  Action Port : ActionPort  ActionPortLabel=elseif(u1 >= 1.575)
  LUT 1.58RR : Lookup_n-D  NumberOfTableDimensions=1  BreakpointsForDimension1=[399.777;506.9266;603.8102;700.5298;796.9731;893.2068;989.2892;1085.262;1181.153;1276.983;1372.766;1468.512;1564.23;1659.923;1755.597;1851.256;1946.9]  Table=[400;500;600;700;800;900;1000;1100;1200;1300;1400;1500;1600;1700;1800;1900;2000]  InternalRulePriority=Speed  RndMeth=Simplest
  Out1 : Outport
  wires:
  In1/1 -> LUT 1.58RR/1
  LUT 1.58RR/1 -> Out1/1

== system LUT_liver_pancreas_25/If Action Subsystem6/If Action Subsystem2/If Action Subsystem6/If Action Subsystem9 ==
  In1 : Inport
  Action Port : ActionPort  ActionPortLabel=if(u1 >= 1.585)
  LUT 1.59RR : Lookup_n-D  NumberOfTableDimensions=1  BreakpointsForDimension1=[399.7377;506.8737;603.7411;700.4391;796.857;893.0624;989.1145;1085.055;1180.913;1276.71;1372.458;1468.169;1563.851;1659.508;1755.147;1850.768;1946.377]  Table=[400;500;600;700;800;900;1000;1100;1200;1300;1400;1500;1600;1700;1800;1900;2000]  InternalRulePriority=Speed  RndMeth=Simplest
  Out1 : Outport
  wires:
  In1/1 -> LUT 1.59RR/1
  LUT 1.59RR/1 -> Out1/1

== system LUT_liver_pancreas_25/If Action Subsystem6/If Action Subsystem2/If Action Subsystem7/If Action Subsystem1 ==
  In1 : Inport
  Action Port : ActionPort  ActionPortLabel=elseif( u1 >= 1.715)
  LUT 1.72RR : Lookup_n-D  NumberOfTableDimensions=1  BreakpointsForDimension1=[399.2669;506.2623;602.9584;699.4192;795.5504;891.4324;987.1341;1082.704;1178.177;1273.576;1368.918;1464.216;1559.478;1654.712;1749.923;1845.114;1940.289]  Table=[400;500;600;700;800;900;1000;1100;1200;1300;1400;1500;1600;1700;1800;1900;2000]  InternalRulePriority=Speed  RndMeth=Simplest
  Out1 : Outport
  wires:
  In1/1 -> LUT 1.72RR/1
  LUT 1.72RR/1 -> Out1/1

== system LUT_liver_pancreas_25/If Action Subsystem6/If Action Subsystem2/If Action Subsystem7/If Action Subsystem10 ==
  In1 : Inport
  Action Port : ActionPort  ActionPortLabel=elseif( u1>= 1.705)
  LUT 1.71RR : Lookup_n-D  NumberOfTableDimensions=1  BreakpointsForDimension1=[399.3007;506.3047;603.0117;699.4881;795.6386;891.5429;987.2688;1082.865;1178.365;1273.791;1369.162;1464.489;1559.781;1655.045;1750.286;1845.508;1940.714]  Table=[400;500;600;700;800;900;1000;1100;1200;1300;1400;1500;1600;1700;1800;1900;2000]  InternalRulePriority=Speed  RndMeth=Simplest
  Out1 : Outport
  wires:
  In1/1 -> LUT 1.71RR/1
  LUT 1.71RR/1 -> Out1/1

== system LUT_liver_pancreas_25/If Action Subsystem6/If Action Subsystem2/If Action Subsystem7/If Action Subsystem2 ==
  In1 : Inport
  Action Port : ActionPort  ActionPortLabel=else
  LUT 1.70RR : Lookup_n-D  NumberOfTableDimensions=1  BreakpointsForDimension1=[399.3349;506.3479;603.066;699.5585;795.7288;891.6556;987.4063;1083.029;1178.556;1274.011;1369.411;1464.767;1560.089;1655.384;1750.655;1845.908;1941.145]  Table=[400;500;600;700;800;900;1000;1100;1200;1300;1400;1500;1600;1700;1800;1900;2000]  InternalRulePriority=Speed  RndMeth=Simplest
  Out1 : Outport
  wires:
  In1/1 -> LUT 1.70RR/1
  LUT 1.70RR/1 -> Out1/1

== system LUT_liver_pancreas_25/If Action Subsystem6/If Action Subsystem2/If Action Subsystem7/If Action Subsystem3 ==
  In1 : Inport
  Action Port : ActionPort  ActionPortLabel=elseif( u1 >= 1.725)
  LUT 1.73RR : Lookup_n-D  NumberOfTableDimensions=1  BreakpointsForDimension1=[399.2335;506.2205;602.9062;699.3518;795.4639;891.3242;987.002;1082.547;1177.993;1273.364;1368.678;1463.947;1559.18;1654.385;1749.565;1844.727;1939.872]  Table=[400;500;600;700;800;900;1000;1100;1200;1300;1400;1500;1600;1700;1800;1900;2000]  InternalRulePriority=Speed  RndMeth=Simplest
  Out1 : Outport
  wires:
  In1/1 -> LUT 1.73RR/1
  LUT 1.73RR/1 -> Out1/1

== system LUT_liver_pancreas_25/If Action Subsystem6/If Action Subsystem2/If Action Subsystem7/If Action Subsystem4 ==
  In1 : Inport
  Action Port : ActionPort  ActionPortLabel=elseif( u1 >= 1.735)
  LUT 1.74RR : Lookup_n-D  NumberOfTableDimensions=1  BreakpointsForDimension1=[399.2004;506.1794;602.855;699.2857;795.3793;891.2182;986.8726;1082.392;1177.812;1273.157;1368.443;1463.683;1558.887;1654.062;1749.214;1844.345;1939.46]  Table=[400;500;600;700;800;900;1000;1100;1200;1300;1400;1500;1600;1700;1800;1900;2000]  InternalRulePriority=Speed  RndMeth=Simplest
  Out1 : Outport
  wires:
  In1/1 -> LUT 1.74RR/1
  LUT 1.74RR/1 -> Out1/1

== system LUT_liver_pancreas_25/If Action Subsystem6/If Action Subsystem2/If Action Subsystem7/If Action Subsystem5 ==
  In1 : Inport
  Action Port : ActionPort  ActionPortLabel=elseif( u1 >= 1.755)
  LUT 1.76RR : Lookup_n-D  NumberOfTableDimensions=1  BreakpointsForDimension1=[399.1352;506.0992;602.7556;699.1577;795.2153;891.0127;986.6214;1082.092;1177.461;1272.752;1367.984;1463.169;1558.316;1653.434;1748.527;1843.6;1938.657]  Table=[400;500;600;700;800;900;1000;1100;1200;1300;1400;1500;1600;1700;1800;1900;2000]  InternalRulePriority=Speed  RndMeth=Simplest
  Out1 : Outport
  wires:
  In1/1 -> LUT 1.76RR/1
  LUT 1.76RR/1 -> Out1/1

== system LUT_liver_pancreas_25/If Action Subsystem6/If Action Subsystem2/If Action Subsystem7/If Action Subsystem6 ==
  In1 : Inport
  Action Port : ActionPort  ActionPortLabel=elseif( u1 >= 1.745)
  LUT 1.75RR : Lookup_n-D  NumberOfTableDimensions=1  BreakpointsForDimension1=[399.1676;506.139;602.8048;699.221;795.2964;891.1144;986.7457;1082.241;1177.635;1272.952;1368.211;1463.424;1558.599;1653.746;1748.868;1843.97;1939.055]  Table=[400;500;600;700;800;900;1000;1100;1200;1300;1400;1500;1600;1700;1800;1900;2000]  InternalRulePriority=Speed  RndMeth=Simplest
  Out1 : Outport
  wires:
  In1/1 -> LUT 1.75RR/1
  LUT 1.75RR/1 -> Out1/1

== system LUT_liver_pancreas_25/If Action Subsystem6/If Action Subsystem2/If Action Subsystem7/If Action Subsystem7 ==
  In1 : Inport
  Action Port : ActionPort  ActionPortLabel=elseif( u1 >= 1.765)
  LUT 1.77RR : Lookup_n-D  NumberOfTableDimensions=1  BreakpointsForDimension1=[399.1032;506.0601;602.7073;699.0957;795.1359;890.9131;986.4995;1081.947;1177.29;1272.555;1367.76;1462.918;1558.038;1653.127;1748.192;1843.237;1938.264]  Table=[400;500;600;700;800;900;1000;1100;1200;1300;1400;1500;1600;1700;1800;1900;2000]  InternalRulePriority=Speed  RndMeth=Simplest
  Out1 : Outport
  wires:
  In1/1 -> LUT 1.77RR/1
  LUT 1.77RR/1 -> Out1/1

== system LUT_liver_pancreas_25/If Action Subsystem6/If Action Subsystem2/If Action Subsystem7/If Action Subsystem8 ==
  In1 : Inport
  Action Port : ActionPort  ActionPortLabel=elseif(u1 >= 1.775)
  LUT 1.78RR : Lookup_n-D  NumberOfTableDimensions=1  BreakpointsForDimension1=[399.0715;506.0216;602.66;699.035;795.0582;890.8156;986.3801;1081.804;1177.123;1272.362;1367.541;1462.671;1557.764;1652.826;1747.863;1842.879;1937.878]  Table=[400;500;600;700;800;900;1000;1100;1200;1300;1400;1500;1600;1700;1800;1900;2000]  InternalRulePriority=Speed  RndMeth=Simplest
  Out1 : Outport
  wires:
  In1/1 -> LUT 1.78RR/1
  LUT 1.78RR/1 -> Out1/1

== system LUT_liver_pancreas_25/If Action Subsystem6/If Action Subsystem2/If Action Subsystem7/If Action Subsystem9 ==
  In1 : Inport
  Action Port : ActionPort  ActionPortLabel=if(u1 >= 1.785)
  LUT 1.79RR : Lookup_n-D  NumberOfTableDimensions=1  BreakpointsForDimension1=[399.0401;505.9837;602.6136;698.9756;794.9821;890.72;986.263;1081.664;1176.958;1272.173;1367.325;1462.429;1557.495;1652.529;1747.539;1842.527;1937.497]  Table=[400;500;600;700;800;900;1000;1100;1200;1300;1400;1500;1600;1700;1800;1900;2000]  InternalRulePriority=Speed  RndMeth=Simplest
  Out1 : Outport
  wires:
  In1/1 -> LUT 1.79RR/1
  LUT 1.79RR/1 -> Out1/1

== system LUT_liver_pancreas_25/If Action Subsystem6/If Action Subsystem2/If Action Subsystem8/If Action Subsystem1 ==
  In1 : Inport
  Action Port : ActionPort  ActionPortLabel=elseif( u1 >= 1.815)
  LUT 1.82RR : Lookup_n-D  NumberOfTableDimensions=1  BreakpointsForDimension1=[398.948;505.8734;602.4798;698.8047;794.7633;890.4452;985.9258;1081.259;1176.483;1271.624;1366.701;1461.727;1556.714;1651.668;1746.597;1841.503;1936.391]  Table=[400;500;600;700;800;900;1000;1100;1200;1300;1400;1500;1600;1700;1800;1900;2000]  InternalRulePriority=Speed  RndMeth=Simplest
  Out1 : Outport
  wires:
  In1/1 -> LUT 1.82RR/1
  LUT 1.82RR/1 -> Out1/1

== system LUT_liver_pancreas_25/If Action Subsystem6/If Action Subsystem2/If Action Subsystem8/If Action Subsystem10 ==
  In1 : Inport
  Action Port : ActionPort  ActionPortLabel=elseif( u1>= 1.805)
  LUT 1.81RR : Lookup_n-D  NumberOfTableDimensions=1  BreakpointsForDimension1=[398.9784;505.9096;602.5235;698.8604;794.8347;890.5349;986.0359;1081.391;1176.638;1271.803;1366.905;1461.957;1556.97;1651.951;1746.906;1841.839;1936.754]  Table=[400;500;600;700;800;900;1000;1100;1200;1300;1400;1500;1600;1700;1800;1900;2000]  InternalRulePriority=Speed  RndMeth=Simplest
  Out1 : Outport
  wires:
  In1/1 -> LUT 1.81RR/1
  LUT 1.81RR/1 -> Out1/1

== system LUT_liver_pancreas_25/If Action Subsystem6/If Action Subsystem2/If Action Subsystem8/If Action Subsystem2 ==
  In1 : Inport
  Action Port : ActionPort  ActionPortLabel=else
  LUT 1.80RR : Lookup_n-D  NumberOfTableDimensions=1  BreakpointsForDimension1=[399.0091;505.9463;602.5681;698.9174;794.9076;890.6265;986.1483;1081.526;1176.797;1271.986;1367.113;1462.191;1557.23;1652.238;1747.219;1842.18;1937.123]  Table=[400;500;600;700;800;900;1000;1100;1200;1300;1400;1500;1600;1700;1800;1900;2000]  InternalRulePriority=Speed  RndMeth=Simplest
  Out1 : Outport
  wires:
  In1/1 -> LUT 1.80RR/1
  LUT 1.80RR/1 -> Out1/1

== system LUT_liver_pancreas_25/If Action Subsystem6/If Action Subsystem2/If Action Subsystem8/If Action Subsystem3 ==
  In1 : Inport
  Action Port : ActionPort  ActionPortLabel=elseif( u1 >= 1.825)
  LUT 1.83RR : Lookup_n-D  NumberOfTableDimensions=1  BreakpointsForDimension1=[398.9179;505.8378;602.4369;698.7501;794.6935;890.3573;985.8178;1081.13;1176.33;1271.447;1366.5;1461.501;1556.462;1651.391;1746.293;1841.172;1936.034]  Table=[400;500;600;700;800;900;1000;1100;1200;1300;1400;1500;1600;1700;1800;1900;2000]  InternalRulePriority=Speed  RndMeth=Simplest
  Out1 : Outport
  wires:
  In1/1 -> LUT 1.83RR/1
  LUT 1.83RR/1 -> Out1/1

== system LUT_liver_pancreas_25/If Action Subsystem6/If Action Subsystem2/If Action Subsystem8/If Action Subsystem4 ==
  In1 : Inport
  Action Port : ActionPort  ActionPortLabel=elseif( u1 >= 1.835)
  LUT 1.84RR : Lookup_n-D  NumberOfTableDimensions=1  BreakpointsForDimension1=[398.8881;505.8028;602.3948;698.6967;794.6252;890.2713;985.7121;1081.002;1176.181;1271.274;1366.302;1461.279;1556.215;1651.117;1745.993;1840.847;1935.682]  Table=[400;500;600;700;800;900;1000;1100;1200;1300;1400;1500;1600;1700;1800;1900;2000]  InternalRulePriority=Speed  RndMeth=Simplest
  Out1 : Outport
  wires:
  In1/1 -> LUT 1.84RR/1
  LUT 1.84RR/1 -> Out1/1

== system LUT_liver_pancreas_25/If Action Subsystem6/If Action Subsystem2/If Action Subsystem8/If Action Subsystem5 ==
  In1 : Inport
  Action Port : ActionPort  ActionPortLabel=elseif( u1 >= 1.855)
  LUT 1.86RR : Lookup_n-D  NumberOfTableDimensions=1  BreakpointsForDimension1=[398.8294;505.7343;602.3132;698.5932;794.4928;890.1047;985.5069;1080.756;1175.89;1270.937;1365.918;1460.846;1555.732;1650.584;1745.409;1840.211;1934.994]  Table=[400;500;600;700;800;900;1000;1100;1200;1300;1400;1500;1600;1700;1800;1900;2000]  InternalRulePriority=Speed  RndMeth=Simplest
  Out1 : Outport
  wires:
  In1/1 -> LUT 1.86RR/1
  LUT 1.86RR/1 -> Out1/1

== system LUT_liver_pancreas_25/If Action Subsystem6/If Action Subsystem2/If Action Subsystem8/If Action Subsystem6 ==
  In1 : Inport
  Action Port : ActionPort  ActionPortLabel=elseif( u1 >= 1.845)
  LUT 1.85RR : Lookup_n-D  NumberOfTableDimensions=1  BreakpointsForDimension1=[398.8586;505.7683;602.3536;698.6444;794.5583;890.1871;985.6084;1080.878;1176.034;1271.104;1366.108;1461.06;1555.971;1650.849;1745.699;1840.527;1935.336]  Table=[400;500;600;700;800;900;1000;1100;1200;1300;1400;1500;1600;1700;1800;1900;2000]  InternalRulePriority=Speed  RndMeth=Simplest
  Out1 : Outport
  wires:
  In1/1 -> LUT 1.85RR/1
  LUT 1.85RR/1 -> Out1/1

== system LUT_liver_pancreas_25/If Action Subsystem6/If Action Subsystem2/If Action Subsystem8/If Action Subsystem7 ==
  In1 : Inport
  Action Port : ActionPort  ActionPortLabel=elseif( u1 >= 1.865)
  LUT 1.87RR : Lookup_n-D  NumberOfTableDimensions=1  BreakpointsForDimension1=[398.8005;505.7008;602.2735;698.5431;794.4288;890.0239;985.4074;1080.636;1175.748;1270.773;1365.731;1460.635;1555.496;1650.324;1745.124;1839.901;1934.658]  Table=[400;500;600;700;800;900;1000;1100;1200;1300;1400;1500;1600;1700;1800;1900;2000]  InternalRulePriority=Speed  RndMeth=Simplest
  Out1 : Outport
  wires:
  In1/1 -> LUT 1.87RR/1
  LUT 1.87RR/1 -> Out1/1

== system LUT_liver_pancreas_25/If Action Subsystem6/If Action Subsystem2/If Action Subsystem8/If Action Subsystem8 ==
  In1 : Inport
  Action Port : ActionPort  ActionPortLabel=elseif(u1 >= 1.875)
  LUT 1.88RR : Lookup_n-D  NumberOfTableDimensions=1  BreakpointsForDimension1=[398.7719;505.6679;602.2346;698.4941;794.3661;889.9449;985.31;1080.518;1175.61;1270.612;1365.547;1460.427;1555.265;1650.068;1744.843;1839.595;1934.328]  Table=[400;500;600;700;800;900;1000;1100;1200;1300;1400;1500;1600;1700;1800;1900;2000]  InternalRulePriority=Speed  RndMeth=Simplest
  Out1 : Outport
  wires:
  In1/1 -> LUT 1.88RR/1
  LUT 1.88RR/1 -> Out1/1

== system LUT_liver_pancreas_25/If Action Subsystem6/If Action Subsystem2/If Action Subsystem8/If Action Subsystem9 ==
  In1 : Inport
  Action Port : ActionPort  ActionPortLabel=if(u1 >= 1.885)
  LUT 1.89RR : Lookup_n-D  NumberOfTableDimensions=1  BreakpointsForDimension1=[398.7436;505.6354;602.1965;698.4461;794.3048;889.8676;985.2145;1080.403;1175.474;1270.454;1365.366;1460.223;1555.037;1649.816;1744.567;1839.294;1934.002]  Table=[400;500;600;700;800;900;1000;1100;1200;1300;1400;1500;1600;1700;1800;1900;2000]  InternalRulePriority=Speed  RndMeth=Simplest
  Out1 : Outport
  wires:
  In1/1 -> LUT 1.89RR/1
  LUT 1.89RR/1 -> Out1/1
